simulink model "rti1401_program_controls_2018_test"  (R2017b)
settings: Solver=ode1  StartTime=0.0  StopTime=Inf  FixedStep=0.001  RelTol=1e-3  EnableMultiTasking=on
PreLoadFcn:
  | dataCar
  | load_vars
  | structAero
  | structEstimPar
  | structSensors
  | structSettings
PostLoadFcn:
  | , if any(exist('dsrtsu_mdlpostloadfcn', 'file') == [2, 3, 6]), try dsrtsu_mdlpostloadfcn('Execute', bdroot); catch fprintf('Error in PostLoadFcn (dsrtsu_mdlpostloadfcn) for model "%s":\n %s\n', bdroot, lasterr); end, end,
InitFcn:
  | dataCar
  | load_vars
  | structAero
  | structEstimPar
  | structSensors
  | structSettings
StartFcn:
  | dataCar
  | load_vars
  | structAero
  | structEstimPar
  | structSensors
  | structSettings
values from neighbouring files (symbols this model uses):
  Throttle_limits = [0.15, 0.90, 0.16, 0.92]    [load_vars.m]
undefined symbols (not defined in the file or in its folder): car, sensors
libraries: rtican x44, hdlsllib x32, simulink x8, rti1401lib_II_base x1
(part 11 of 11)

== matlab function rti1401_program_controls_2018_test/Processor/Control Systems/Traction Control ==
  data: sensors input; Torques output; settings input; estimPar input; torqueDistribution input; slipSet input; car parameter; TiTi2 output; error output; rpmSet output
function [Torques, TiTi2, error, rpmSet] = Traction(sensors, settings, estimPar, torqueDistribution, slipSet, car)

error =[0 0 0 0]';
persistent errorInt; if isempty(errorInt); errorInt=[0 0 0 0]'; end
persistent errorD; if isempty(errorD); errorD=[0 0 0 0]'; end
persistent errorPrev; if isempty(errorPrev); errorPrev=[0 0 0 0]'; end

%persistent wi_prev; if isempty(wi_prev); wi_prev=[0 0 0 0]'; end
%persistent SR_expected; if isempty(SR_expected); SR_expected=zeros(4, 8); end
%persistent wvi_prev; if isempty(wvi_prev); wvi_prev=[0 0 0 0]'; end

persistent TiPrev; if isempty(TiPrev); TiPrev=[0 0 0 0]'; end

persistent errorInt2; if isempty(errorInt2); errorInt2=[0 0 0 0]'; end
persistent Ti; if isempty(Ti); Ti=[0 0 0 0]'; end
persistent Ti2; if isempty(Ti2); Ti2=[0 0 0 0]'; end

rpmSet = [20000;20000;20000;20000];

if settings.TC == 1

    slipRatioTarget = slipSet;
    dist = estimPar.Fzi/sum(estimPar.Fzi);
    
    Kp = 100*dist*10;
    Ki = 40*dist*1000;
    Kd = 0*dist/100;
    Kv = 70/100;
    Mu = car.mu;
    
    Kp2 = 20*dist/1000;
    Ki2 = 40*dist/1000;
    
    %normal non linear torque control
    error = slipRatioTarget - estimPar.slip;
    
    errorInt = errorInt + error*car.dt;
    errorInt = min(max(errorInt,-0.001*[1;1;1;1]),0.003*[1;1;1;1]);
    errorD = min(max(errorD*0.1 + 0.9*(error - errorPrev)/car.dt,-25),25);
    lambdaD = Kp.*error + Ki.*errorInt + Kd.*errorD;
    Ti = lambdaD*car.tireInertia*max(estimPar.v,0)^Kv/car.tireRadius + sign(torqueDistribution).*estimPar.Fzi*(Mu)*car.tireRadius;
    Ti = Ti / car.gearRatio;
    
    %optimum seeking
    dFds = dFdsCalculator(estimPar.Fxi,estimPar.slip);
    error2 = dFds - 0;
    errorInt2 = errorInt2 + error2*car.dt;
    errorInt2 = min(max(errorInt2,-500*[1;1;1;1]),500*[1;1;1;1]);
    lambdaD2 = Kp2.*error2 + Ki2.*errorInt2;
    Ti2 = lambdaD2*car.tireInertia*max(estimPar.v,0)^Kv/car.tireRadius + sign(torqueDistribution).*estimPar.Fzi*(car.TC_mu)*car.tireRadius;
    Ti2 = Ti2 / car.gearRatio;
    
    for i=1:4
        if abs(error(i)) < 0.05
            Ti(i) = Ti2(i);
        end
    end
    
    if estimPar.v < 1/3.6
        %Ti = [80 80 180 180]';
        errorInt = [0 0 0 0]';
    end

    if sensors.throttle < 0.1
        errorInt = [0 0 0 0]';
    end
    
    lowerBoundary = TiPrev - 100/car.gearRatio;
    upperBoundary = TiPrev + 100/car.gearRatio;

    Ti = min(max(Ti,lowerBoundary),upperBoundary);
    
    TiPrev = Ti;
    errorPrev = error;
    
    Torques = Ti;
    for i=1:4
        if torqueDistribution(i) > 0
            Torques(i) = max(min(Torques(i),torqueDistribution(i)),0); 
        else
            Torques(i) = min(max(Torques(i),torqueDistribution(i)),0);
        end
    end
    
    
else
    Torques = torqueDistribution;
end

checkTorquemax = find((Torques > car.motor.Tmax)==1); %Limit torques to max torque
Torques(checkTorquemax)=car.motor.Tmax(checkTorquemax);



%wi_prev = sensors.wheelspeed;
%wvi_prev = sensors.wheelspeedi;

TiTi2 = [Ti;Ti2];

end

function [dFds] = dFdsCalculator(Fx,slipRatio)
N = 6;

persistent slipVector, if isempty(slipVector); slipVector = zeros(N,4); end
persistent FxVector, if isempty(FxVector); FxVector = zeros(N,4); end


FxVector(1,:) = Fx;
slipVector(1,:) = slipRatio;

dFds = [0;0;0;0];

for i=1:4
    p1 = polyfit(slipVector(:,i),FxVector(:,i),1);
    p2 = polyfit(FxVector(:,i),slipVector(:,i),1);
    
    rico1 = p1(1);
    rico2 = 1/p2(1);
    
    rico = sign(min(abs(rico1),abs(rico2)))*min(abs(rico1),abs(rico2));

    dFds(i) = max(min(rico,20000),-20000);
end

% shift list one
dummy = FxVector(1:N-1,:);
FxVector = [[0,0,0,0];dummy];
dummy = slipVector(1:N-1,:);
slipVector = [[0,0,0,0];dummy];

end

== matlab function rti1401_program_controls_2018_test/Processor/Control Systems/Yaw Rate Control ==
  data: sensors input; Mz output; settings input; estimPar input; car parameter; error output; actions output; rref output
function [Mz,error,actions,rref]= yawRateControl(sensors, settings, estimPar, car)
%Function that controls the moment around the z-axis
%INPUTS:
%OUTPUT: Moment of the car around Z-axis [Nm]

Mz = 0;
Mz_temp = 0;
rref = estimPar.rref;
error = 0;

wheelAngle = (sensors.wheelAngles(1)+sensors.wheelAngles(2))/2;

persistent Mz_memory; if isempty(Mz_memory); Mz_memory = 0; end
persistent errorInt; if isempty(errorInt); errorInt = 0; end
persistent errorDev; if isempty(errorDev); errorDev = 0; end
persistent prevError; if isempty(prevError); prevError = 0; end
persistent prevWheelAngle; if isempty(prevWheelAngle); prevWheelAngle = 0; end
persistent prevRref; if isempty(prevRref); prevRref = 0; end


error = estimPar.rref - sensors.yawRate;
errorInt = errorInt + error*car.dt;
errorInt = min(max(errorInt,-car.YRC.intLimit),car.YRC.intLimit);
errorDev = (error - prevError)/car.dt;
wheelAngleDev = (wheelAngle - prevWheelAngle)/car.dt;
rrefDev = (estimPar.rref - prevRref)/car.dt;

velocityGain = min(max(1 - (estimPar.v - car.YRC.changeVelocity)*car.YRC.slope,0),1);

Mz_temp = (car.YRC.Kp*error + car.YRC.Ki*errorInt + car.YRC.Kd*errorDev...
    +car.YRC.Ks*wheelAngleDev + car.YRC.Kr*rrefDev)*velocityGain;
Mz_temp = max(min(Mz_temp,car.YRC.maxValue),-car.YRC.maxValue);
Mz_memory=Mz_memory+Mz_temp;

P_Action = car.YRC.Kp*error;
I_Action = car.YRC.Ki*errorInt;
D_Action = car.YRC.Kd*errorDev;
steeringWheel_Action = car.YRC.Ks*wheelAngle;
yawRate_Action = car.YRC.Kr*estimPar.rref;

actions = [P_Action;I_Action;D_Action;steeringWheel_Action;yawRate_Action];
prevError = error;
prevWheelAngle = wheelAngle;
prevRref = estimPar.rref;



% if settings.YRC == 2
%     error = estimPar.rref - sensors.yawRate;
%     integral = integral + error*car.dt;
%     derivative = (error - prevError)/car.dt;
%
%     Mz_temp = car.YRC.Kp*error + car.YRC.Ki*integral + car.YRC.Kd*derivative...
%         +car.YRC.Ks*wheelAngle + car.YRC.Kr*estimPar.rref;
%     Mz_temp = max(min(Mz_temp,car.YRC.maxValue),-car.YRC.maxValue);
%
%     prevError = error;
% end



if settings.YRC ==1 %YRC enabled
    Mz = Mz_memory;
else %YRC disabled
    Mz = 0;
end

if car.YRC.minV > estimPar.v
    Mz = 0; %if speed is too low, don't activate yaw rate control
    errorInt = 0;
    prevError = 0;
end

rref=estimPar.rref;

== matlab function rti1401_program_controls_2018_test/Processor/Controller Settings1 ==
  data: settings output Bus: settingBus; sensors input; torqueMode input; Fsens input; TC input; Power input; Regen input; unlimitedFx input; effEstimation input; YRC input
function settings  = settingController(sensors,torqueMode,Fsens,TC,Power,Regen,unlimitedFx,effEstimation,YRC)

%TODO in test: bypass met P_elec controle, altijd tenzij P_elec sensor niet werkt

%==============%
%   Options    %
% 1 settings.torqueMode : 0,1,2
% 2 settings.Fsens : 0-100 in steps of 5
% 3 settings.TC : 0 or 1 (on/off)
% 4 settings.Power : 0-100 in steps of 10
% 5 settings.Regen : 0-30 in steps of 5
% 6 settings.unlimitedFx : 0 of 1
% 7 settings.effEstimation : 0,1,2
% 8 settings.YRC : 0 or 1 (on/off)
%==============%

error_detection = 1;
if any(sensors.errors == error_detection)
    if any(sensors.TCRE == error_detection)
        TC = 0;
    end
    torqueMode = uint8(0);
end

settings.Fxsens = 1;
settings.torqueMode = double(torqueMode);
settings.Fsens = double(Fsens);
settings.TC = TC;
settings.Power = double(Power)/16;
settings.Regen = double(Regen);
settings.unlimitedFx = unlimitedFx;
settings.effEstimation = effEstimation;
settings.YRC = YRC;

== matlab function rti1401_program_controls_2018_test/Processor/Decisive Logic Block/MATLAB Function ==
  data: torqueController input; torques output; rpmController input; torqueBypass input; rpmBypass input; rpmRef output; settings input
function [torques,rpmRef]= DLB(torqueController,rpmController,torqueBypass,rpmBypass,settings)

torques = [0;0;0;0];
rpmRef = [0;0;0;0];

if settings.torqueMode == 0
    
    torques = settings.Power*torqueBypass;
    rpmRef = rpmBypass;
    
else
    
    torques = settings.Power*torqueController;
    rpmRef = rpmController;
    
end

== matlab function rti1401_program_controls_2018_test/Processor/Vehicle Estimated Parameters/Extended Kalman Filter ==
  data: F_KF input; States output; H_KF input; y_meas input; y_pred input; R_beta_lin input; Q_Cy input; sensors input; P_est input; P_est output
function [States, P_est]  = EKF(F_KF,H_KF,y_meas, y_pred, R_beta_lin, Q_Cy, sensors, P_est)
 
 %% Initialization of global variables %%
 
global vy_g psi_dot_g vx_g Cf_g Cr_g P_est_glob

delta = (sensors.wheelAngles(1)+sensors.wheelAngles(2))/2;
 %% Calculation partitioned F-matrix %%
F = F_KF;
 
 %% Calculation partitioned H-matrix %%
H = H_KF;

% ============================== Parameters ===============================
% number of observable states
n_xo = 3;
% number of unobservable states
n_xu = 2;
% total number of states
n_x = n_xo + n_xu;
% number of system inputs
n_u = 2;
% number of measurements
n_y = 7;
% covariance of modeled process noise

Q_Cyf = Q_Cy;
Q_Cyr = Q_Cy;
Q_vy = 1*10^(-6);
Q_psi_dot = 1*10^(-6);
Q_vx = 1*10^(-4);

Q_oo = [Q_vy, 0, 0;
    0, Q_psi_dot, 0;
    0, 0, Q_vx];

Q_uu = [Q_Cyf, 0;
     0, Q_Cyr];
 
Q_model = [Q_vy, 0, 0, 0, 0;
    0, Q_psi_dot, 0, 0, 0;
    0, 0, Q_vx, 0, 0;
    0, 0, 0, Q_Cyf, 0;
    0, 0, 0, 0, Q_Cyr];

% covariance of measurement noise

R_psi_dot = 2.4*10^(-7);
R_ay = 2.5*10^(-3);
R_vxfl = 1*10^(-5);
R_vxfr = 1*10^(-5);
R_vxrl = 1*10^(-5);
R_vxrr = 1*10^(-5);
R_beta = R_beta_lin;
R_model = [R_psi_dot, 0, 0, 0, 0, 0, 0;
    0, R_ay, 0, 0, 0, 0, 0;
    0, 0, R_vxfl, 0, 0, 0, 0;
    0, 0, 0, R_vxfr, 0, 0, 0;
    0, 0, 0, 0, R_vxrl, 0, 0;
    0, 0, 0, 0, 0, R_vxrr, 0;
    0, 0, 0, 0, 0, 0, R_beta];
% covariance of simulated process noise
Q_sim = [Q_vy, 0, 0, 0, 0;
    0, Q_psi_dot, 0, 0, 0;
    0, 0, Q_vx, 0, 0;
    0, 0, 0, Q_Cyf, 0;
    0, 0, 0, 0, Q_Cyr];
% covariance of simulated measurement noise
R_sim = [R_psi_dot, 0, 0, 0, 0, 0, 0;
    0, R_ay, 0, 0, 0, 0, 0;
    0, 0, R_vxfl, 0, 0, 0, 0;
    0, 0, 0, R_vxfr, 0, 0, 0;
    0, 0, 0, 0, R_vxrl, 0, 0;
    0, 0, 0, 0, 0, R_vxrr, 0;
    0, 0, 0, 0, 0, 0, R_beta];
% initial state
x0 = [0; 0; 0; car.Cf_lin; car.Cr_lin];
% initial state estimate
% x_est0 = [0; 0; 0; car.Cf_lin; car.Cr_lin];
% feedback values
% kx = 0.1;
% ky = 0.1;
% kt = 0.1;

% ==================== Simulation Preparation ===========================

if isempty(P_est_glob) == 1
    states = x_0;
    P_est= eye(n_x)*10^(-4);
    
else
    states = [vy_g, psi_dot_g, vx_g, Cf_g, Cr_g];
    
end
       
inputs_EKF = [delta; sensors.ax];

P_est_pre_tot = zeros(n_x, n_x);

P_est_post_tot = zeros(n_x, n_x);


% feedback matrix
% K = [kx,  0,  0;
%       0, ky, kt];


% ==================== Kalman prediction step ===========================

states = f_est(states, inputs_EKF, car.dt);

P_est_pre = F*P_est*F^(-1)+Q_model;

%P_est_pre_oo = A*P_est_post(:,:,i-1)*A' + Q_mod;
%      P_est(:,:,i) = A*P_est(:,:,i-1)*A';

% ==================== Kalman correction step ===========================

nu = y_meas - y_pred;
%      nu(:,i) = y(:,i) - h(x_est(:,i));
S = H*P_est_pre*H' + R_model;
%      S(:,:,i) = C*P_est(:,:,i)*C';
K = P_est_pre*H'/S;

states = states + K*nu;
P_est_post = (eye(n_x)-K*H)*P_est_pre;

States.vy_g = states(1);
States.psi_dot_g = states(2);
States.vx_g = states(3);
States.Cf_g = states(4);
States.Cr_g = states(5);

P_est = P_est_post;
P_est_glob = P_est;

% %     Control law
% u(:,i) = u_ref(:,i);
% %     err_loc(:,i) = local_error(x_ref(:,i), x_est(:,i));
% %     u(:,i) = u_ref(:,i) + K*err_loc(:,i);

end

== matlab function rti1401_program_controls_2018_test/Processor/Vehicle Estimated Parameters/Covariantie ==
  data: sensors input; R_beta_lin output; yawrate_lin input; Q_Cy output; car parameter
function [R_beta_lin, Q_Cy] = Covariantie(sensors,yawrate_lin, car)
if (abs(sensors.yawRate)-abs(yawrate_lin)) > car.e_max && abs(sensors.yawRate)>0 && abs(yawrate_lin)>0
    
    global counter
    
    if isempty(counter)
        counter = 0
    end
    
    counter = counter + 1;
    array_dev_yawrate = zeros(1,1.5*(1/car.dt));
    delta = (sensors.wheelAngles(1)+sensors.wheelAngles(2))/2;
    % Q_Cyi wordt hoog gezet, net als R_beta_lin, en hoe groter het verschil, hoe groter de 
    % onnauwkeurigheid zal worden (dev_ya wrate = e uit de paper)
    dev_yawrate = abs(sensors.yawRate)-abs(yawrate_lin);
    
    if counter < 1.5*(1/car.dt)
        array_dev_yawrate(counter) = dev_yawrate;
        
    else
        for k = 2:length(array_dev_yawrate)
            array_dev_yawrate(k-1)=array_dev_yawrate(k);
        end
        array_dev_yawrate(length(array_dev_yawrate)) = dev_yawrate;
    end
    
    dev_yawrate_max = max(array_dev_yawrate);
    % We gaan best een referentiewaarde nemen voor Q_Cyi voor het geval het
    % verschil < car.e_max
    Q_Cy0 = car.Q_Cyref*log(9*(delta/car.delta_max)+1);%functie nog aanpasbaar
    R_beta_lin0 = car.R_beta_linref*log(8*(delta/car.delta_max)+2);
    
    
    
    Q_Cy = Q_Cy0 + 500*dev_yawrate_max^2;
    R_beta_lin = R_beta_lin0 + (5*array_dev_yawrate)^4;
    
else
    delta = (sensors.wheelAngles(1)+sensors.wheelAngles(2))/2;
    Q_Cy0 = car.Q_Cyref*log(9*(delta/car.delta_max)+1);%functie nog aanpasbaar
    R_beta_lin0 = car.R_beta_linref*log(8*(delta/car.delta_max)+2);
    Q_Cy = Q_Cy0;
    R_beta_lin = R_beta_lin0;
end

end

== matlab function rti1401_program_controls_2018_test/Processor/Vehicle Estimated Parameters/Estimation Parameters ==
  data: States input; estimPar output; car parameter; sensors parameter; Fzi input; Fyi input; Fxi input; alpha input; eff input; rref input
function estimPar  = estimation_par(States, car, sensors, Fzi, Fyi, Fxi, alpha, eff, rref)
%% Forming "States_final" %%

estimPar.vy_g = States.vy_g;
estimPar.psi_dot_g = States.psi_dot_g;
estimPar.vx_g = States.vx_g;
estimPar.Cf_g = States.Cf_g;
estimPar.Cr_g = States.Cr_g;
estimPar.Fzi=Fzi;
estimPar.Fxi=Fxi;
estimPar.Fyi=Fyi;
estimPar.alpha_f = alpha.f;
estimPar.alpha_r = alpha.r;
estimPar.eff = eff;
estimPar.rref = rref;
end

== matlab function rti1401_program_controls_2018_test/Processor/Vehicle Estimated Parameters/Fx_estimation ==
  data: States input; Fxi output; car parameter; sensors parameter
function Fxi  = Fx_estimation(States,car, sensors)

%OPM: gearratio zit al verwerkt in sensors.torque (= wheelTorque)

persistent wheelspeedPrev; if isempty(wheelspeedPrev); wheelspeedPrev = [0 ;0 ;0 ;0]; end
persistent inertia; if isempty(inertia); inertia = car.tireInertia; end
if isempty(States.vx_g); States.vx_g =0;end
wheelspeed = sensors.wheelspeed;
alpha = (wheelspeed - wheelspeedPrev)/car.dt;

%wheelTorque = car.gearRatio*sensors.torque -(car.motor.Inertia*car.gearRatio^2 - car.tireInertia)*alpha;
%to be used if only motor torque is known (real scenario)

%Fxi_est = (wheelTorque - alpha*inertia)/car.tireRadius;
Fxi_est = (sensors.torque - alpha*inertia)/car.tireRadius;
%Fxi_est = (sensors.torque)/car.tireRadius;

Fx_tot = sensors.ax*car.mass + 0.5*car.rhoAir*States.vx_g^2*car.Cd*car.AFront;
Fxi = Fxi_est;




wheelspeedPrev=wheelspeed;
inertiaOut = inertia;
end

== matlab function rti1401_program_controls_2018_test/Processor/Vehicle Estimated Parameters/Fy_distribution ==
  data: States input; Fyi output; car parameter; sensors parameter; Fzi input; alpha output
function [Fyi,alpha] = Fy_distribution(States,car, sensors, Fzi)

%% Calculation sideslip angles of the wheels %%
delta = (sensors.wheelAngles(1)+sensors.wheelAngles(2))/2;
alpha.f = -((States.vy_g + car.lf*States.psi_dot_g)/(States.vx_g)) + delta;
alpha.r = -((States.vy_g - car.lr*States.psi_dot_g)/(States.vx_g));

%% Calculation OF Lateral forces (Bycicle model) %%
F_yf = 2*States.Cf_g*alpha.f;
F_yr = 2*States.Cr_g*alpha.r;

%% Distribution of lateral force on left and right tire by using the normal force distribution %%


%Use of a scale factor 

FzRatioFront = [Fzi(1); Fzi(2)]./sum(Fzi(1:2));
FzRatioRear = [Fzi(3); Fzi(4)]./sum(Fzi(3:4));


scaleFactorFy = 0.7;
FyFrontDiff = (FzRatioFront(1) - FzRatioFront(2))*scaleFactorFy/2;
Fy_FL = F_yf/2 + FyFrontDiff* F_yf;
Fy_FR = F_yf/2 - FyFrontDiff* F_yf;
FyRearDiff = (FzRatioRear(1) - FzRatioRear(2))*scaleFactorFy/2;
Fy_RL = F_yr/2 + FyRearDiff* F_yr;
Fy_RR = F_yr/2 - FyRearDiff* F_yr;
    
Fyi=[Fy_FL;Fy_FR;Fy_RL;Fy_RR];

== matlab function rti1401_program_controls_2018_test/Processor/Vehicle Estimated Parameters/Fz_estimation ==
  data: States input; Fzi output; car parameter; sensors parameter; aero output
function [Fzi, aero] = Fz_estimation(States,car, sensors)

%% Calculation of Normal Forces F_zi %%

if isempty(States.vx_g); States.vx_g =0;end
%Dynamical loads 
%Without taking suspension into account

aero.FD = 0.5*car.Cd*car.AFront*car.rhoAir*States.vx_g^2; %drag force, pointing rearward [N]
aero.FL = 0.5*car.Cl*car.AFront*car.rhoAir*States.vx_g^2; %lift force, pointing upward [N]
aero.lever_FD = [-0.1;0.1]; %distance from the COG to the point of application of the drag [m]
aero.lever_FL = [-0.1;0.1]; %distance from the COG to the point of application of the lift [m]

FFA = car.g*car.mass*car.lr/car.wb - (car.h/car.wb)*(car.mass*sensors.ax) - ...
    aero.FD*((car.h+aero.lever_FD(2))/car.wb) - ...
    aero.FL*((car.lr-aero.lever_FL(1))/car.wb); %dyn load Front Axle
FRA = car.g*car.mass*car.lf/car.wb + (car.h/car.wb)*(car.mass*sensors.ax) + ...
    aero.FD*((car.h+aero.lever_FD(2))/car.wb) - ...
    aero.FL*((car.lf+aero.lever_FL(1))/car.wb); %dyn load Rear Axle


FFL = FFA/2 - (car.h/(2*car.tw))*(car.mass*sensors.ay);
FFR = FFA/2 + (car.h/(2*car.tw))*(car.mass*sensors.ay);
FRL = FRA/2 - (car.h/(2*car.tw))*(car.mass*sensors.ay);
FRR = FRA/2 + (car.h/(2*car.tw))*(car.mass*sensors.ay);


Fzi = [FFL;FFR;FRL;FRR];

== matlab function rti1401_program_controls_2018_test/Processor/Vehicle Estimated Parameters/MATLAB Function ==
  data: eff output; settings input; car parameter; sensors input
function eff = Efficiency(settings,car, sensors)
%P_elec * eff = P_mech

persistent effTemp; if isempty(effTemp); effTemp = 0.7; end
persistent errorInt; if isempty(errorInt); errorInt = 0; end

Pmax = car.Pmax - car.PC.safetyMargin; %[W]

P_mech = sum(sensors.torque.*sensors.wheelspeed); %*car.gearRatio
P_elec = sensors.P_elec;
ratio = 0.2;

if settings.effEstimation == 1
    
    if P_elec > 1
        effCalc = P_mech/P_elec;
        effTemp = effTemp*ratio + (1-ratio)*min(max(effCalc,car.PC.minEff),car.PC.maxEff);
        
    elseif P_elec < 1
        effCalc = P_elec/min(P_mech,-1);
        effTemp = effTemp*ratio + (1-ratio)*min(max(effCalc,car.PC.minEff),car.PC.maxEff);
        
        
        %mogelijkheid tot uitbreiding: Pmax variable ifv van batterij voor tijdens
        %indurance
    end
    
end

if settings.effEstimation == 2
    
    if P_elec > Pmax*0.3 && sensors.throttle > 0 % only positive power limit
        
        error = (Pmax - P_elec)/Pmax;
        if error < 0 % P_elec > Pmax
            error = error*2;
        end
        
        errorInt = errorInt + error*car.dt;
        errorInt = max(min(errorInt,0.2),-0.2);
        
        dEff = car.PC.Kp*error + car.PC.Ki*errorInt; %more fitting variable name would be powerReductionFactor as this is not anymore an efficiency as Pelec * eff = Pmech
        %make car.PC.Kp velocity dependend?
        
        effTemp = max(min(effTemp + dEff,car.PC.maxEff),car.PC.minEff);
        
    else
        if P_elec > 5000
            eta = P_mech/P_elec;
            effTemp = effTemp*ratio+(1-ratio)*min(max(eta,car.PC.minEff),car.PC.maxEff);
        elseif P_elec < -5000
            eta = P_elec/min(P_mech,-1);
            effTemp = effTemp*ratio+(1-ratio)*min(max(eta,car.PC.minEff),car.PC.maxEff);
        end
        
    end
    
else
    effTemp = effTemp;
    
end


eff = effTemp;
effnotcontrolled = P_mech/P_elec;

== matlab function rti1401_program_controls_2018_test/Processor/Tire model//friction coefficient estimation/MATLAB Function ==
  data: mu input; estimParExtended output; estimPar input
function estimParExtended  = estimParExtension(mu, estimPar)

estimParExtended.vy_g = estimPar.vy_g;
estimParExtended.psi_dot_g = estimPar.psi_dot_g;
estimParExtended.vx_g = estimPar.vx_g;
estimParExtended.Cf_g = estimPar.Cf_g;
estimParExtended.Cr_g = estimPar.Cr_g;
estimParExtended.Fzi=estimPar.Fzi;
estimParExtended.Fxi=estimPar.Fxi;
estimParExtended.Fyi=estimPar.Fyi;
estimParExtended.alpha_f = estimPar.alpha.f;
estimParExtended.alpha_r = estimPar.alpha.r;
estimParExtended.eff = estimPar.eff;
estimParExtended.mu = mu;
estimParExtended.rref = estimPar.rref;

== matlab function rti1401_program_controls_2018_test/Processor/Vehicle Estimated Parameters/Slip Ratio ==
  data: States input; slip_ratio output; car parameter; sensors parameter
function slip_ratio = slip_ratio(States, car, sensors)

if isempty(States.vx_g); States.vx_g =0;end
yawRate = [0;0;States.psi_dot_g];
dist = [car.lf   -car.lf   car.lr   -car.lr;
        car.tl/2 -car.tl/2 car.tr/2 -car.tr/2;
        0        0         0        0];
omegaR = sensors.wheelspeed*car.tireRadius;

%Thesis BreyneMeulemans eq 3.20-3.22
v_xcomp = zeros(4,1);
d = sensors.wheelAngles;
for i=1:4
    R = [cos(d(i)) sin(d(i)) 0;
        -sin(d(i)) cos(d(i)) 0;
        0          0         1];
    v_rel = cross(yawRate,dist(:,i));
    v_abs = v_rel + [States.vx_g;0;0];
    v_ab2 = R*v_abs;
    v_xcomp(i) = v_ab2(1);
end

if sensors.ax > 0
    slip_ratio = (omegaR - v_xcomp)./omegaR;
elseif sensors.ax < 0
    slip_ratio = (omegaR - v_xcomp)./v_xcomp;
else
    slip_ratio = [0;0;0;0];
end
end

== matlab function rti1401_program_controls_2018_test/Processor/Vehicle Estimated Parameters/Yawrate Reference ==
  data: rref output; States input; car parameter; sensors parameter
function rref = yawRateRef(States, car, sensors)
if isempty(States.vx_g); States.vx_g =0;end
%Ackermann
wheelAngle = (sensors.wheelAngles(1)+sensors.wheelAngles(2))/2;
rref = wheelAngle*States.vx_g/car.wb;

== matlab function rti1401_program_controls_2018_test/Processor/Vehicle Estimated Parameters/States_matrix_generation ==
  data: estimPar input; States_matrix_front output; N_est input; Fy_est input; Fx_est input; States_matrix_rear output; slip_ratio input
function [States_matrix_front, States_matrix_rear] = States_matrix_gen(estimPar, N_est, Fy_est, Fx_est, slip_ratio)

global counter_mat 

if isempty(counter_mat)
    counter_mat = 0
end

counter_mat = counter_mat+1;
States_matrix_front = zeros(3,1);
States_matrix_rear = zeros(3,1);
slip_ratio_front = (slip_ratio(1)+slip_ratio(2))/2;
slip_ratio_rear = (slip_ratio(3)+slip_ratio(4))/2;

while counter_mat < 1000
    States_matrix_front(:,counter_mat) = [estimPar.alpha_f, N_est.f, Fy_est.f, slip_ratio_front, Fx_est.f];
    States_matrix_rear(:,counter_mat) = [estimPar.alpha_r, N_est.r, Fy_est.r, slip_ratio_rear, Fx_est.r];
    
end
end

== matlab function rti1401_program_controls_2018_test/Processor/Vehicle Estimated Parameters/Normal forces calculation ==
  data: States input; N_est output; Fy_est output; car parameter; sensors parameter; Fxi input; Fx_est output
function [N_est, Fy_est, Fx_est] = N_F_calc(States, car, sensors, Fxi)

N_est.f = (car.mass)*9.81*((car.lr)/(car.lr+car.lf))- (sensors.ax)*(car.mass)*(car.h);
N_est.r = (car.mass)*9.81*((car.lr)/(car.lr+car.lf))+ (sensors.ax)*(car.mass)*(car.h);

Fy_est.f = 2*(States.Cf_g)*(alpha.f);
Fy_est.r = 2*(States.Cf_r)*(alpha.r);

Fx_est.f = Fxi(1)+Fxi(2);
Fx_est.r = Fxi(3)+Fxi(4);

== matlab function rti1401_program_controls_2018_test/Processor/Vehicle Estimated Parameters/MATLAB Function1 ==
  data: States input; alpha_wheels output; sensors parameter; car parameter
function alpha_wheels  = v_alpha_decomp(States, sensors, car)

%% Calculation vx on each independant wheel %%

vx_wheels.fl = (States.vx_g - States.psi_dot_g*(car.tf/2))*cos(sensors.wheelAngles(1)) + ...
        States.psi_dot_g*(car.lf)*sin(sensors.wheelAngles(1));
    
vx_wheels.fr = (States.vx_g + States.psi_dot_g*(car.tf/2))*cos(sensors.wheelAngles(2)) + ...
        States.psi_dot_g*(car.lf)*sin(sensors.wheelAngles(2));
    
vx_wheels.rl = (States.vx_g - States.psi_dot_g*(car.tr/2));
    
vx_wheels.rr = (States.vx_g + States.psi_dot_g*(car.tr/2));

%% Calculation vy on each independant wheel %%

vy_wheels.fl = (States.vy_g + States.psi_dot_g*(car.lf))*cos(sensors.wheelAngles(1)) + ...
        States.psi_dot_g*(car.tf/2)*sin(sensors.wheelAngles(1));
    
vy_wheels.fr = (States.vy_g - States.psi_dot_g*(car.tf/2))*sin(sensors.wheelAngles(2)) + ...
        States.psi_dot_g*(car.lf)*cos(sensors.wheelAngles(2));
    
vy_wheels.rl = (States.vy_g - States.psi_dot_g*(car.lr));
    
vy_wheels.rr = (States.vy_g - States.psi_dot_g*(car.lr));

%% Calculation alpha's on each independant wheel %%

alpha_wheels.fl = atan2(vy_wheels.fl,vx_wheels.fl);
alpha_wheels.fr = atan2(vy_wheels.fr,vx_wheels.fr);
alpha_wheels.rl = atan2(vy_wheels.rl,vx_wheels.rl);
alpha_wheels.rr = atan2(vy_wheels.rr,vx_wheels.rr);

== matlab function rti1401_program_controls_2018_test/Processor/Tire model//friction coefficient estimation/Tire model estimation ==
  data: States_matrix_front input; Settings_extended output; States_matrix_rear input; Settings input; Magic_tire_param output
function [Settings_extended, Magic_tire_param] ...
    = Est_tire_model(States_matrix_front, States_matrix_rear, Settings)


if length(States_matrix_front) == 1000   % Indien we sampelen op 100Hz krijgen we dit in 10s
                                         % wat ongeveer de duur is van het
                                         % skidpad event
    p0 = tire_model_est_test(States_matrix_front, States_matrix_rear);
    Settings.act_TV = 1;
end

% The following if-statement is ONLY used when the tire model is
% determined. In the normal case, the driver decides wheter or not he
% activates the TV-mode. When the tire model will be determined (probably
% during skidpad event), following if-statement simply overrules the
% decision of the driver. This means, in the first run of the skidpad
% event, the driver won't be able to use the TV-mode.

if length(States_matrix_front) > 1000
    Settings.torqueMode = 1;
else
    Settings.torqueMode = 0;
end

Settings_extended = Settings;
Magic_tire_param.front_x = p0.front_x;
Magic_tire_param.front_y = p0.front_y;
Magic_tire_param.rear_x = p0.rear_x;
Magic_tire_param.rear_y = p0.rear_y;

== matlab function rti1401_program_controls_2018_test/Processor/Tire model//friction coefficient estimation/friction frank test   ==
  data: mu output; estimPar input; Magic_tire_param input; Fzi input; slip_ratio input; alpha_wheels input; States_matrix_front input
function mu  = frictionfrank(estimPar,Magic_tire_param,Fzi,slip_ratio, alpha_wheels, States_matrix_front)
%This function calculates an estimate for the maximum friction coefficient
%by comparing the estimated forces with the forces calculated using the
%Dugoff tire model for a certain side slip angle and slip ratio. The forces
%are calculated for a range of mu values, and the mu for which the forces
%deviate the least (rms) is chosen as the instantaneous mu value.
if length(States_matrix_front) >= 1000
    mu = [0.05;0.05;0.05;0.05];
    rms1 = [0;0;0;0];
    rms2 = [0;0;0;0];

    alpha_mu = [alpha_wheels.fl, alpha_wheels.fr, alpha_wheels.rl, alpha_wheels.rr];

    p0x = [Magic_tire_param.front_x; Magic_tire_param.front_x; ...
    Magic_tire_param.rear_x;Magic_tire_param.rear_x];
    p0y = [Magic_tire_param.front_y; Magic_tire_param.front_y; ...
        Magic_tire_param.rear_y;Magic_tire_param.rear_y];

    for i=1:1:4
        F_xd = Fzi(i)*p0x(i,3)*sin(p0x(i,2)*atan(p0x(i,1)*(1-p0x(i,4))*slip_ratio(i) + ...
            atan(p0x(i,1)*slip_ratio(i))));
        F_yd = Fzi(i)*p0y(i,3)*sin(p0y(i,2)*atan(p0y(i,1)*(1-p0y(i,4))*alpha_mu(i) + ...
            atan(p0y(i,1)*alpha_mu(i))));
   
        rms1(i) = sqrt((estimPar.Fxi(i)-F_xd)^2+(estimPar.Fyi(i)-F_yd)^2);
    end
    for i=1:1:4
        for mu1=0.1:0.05:1
            F_xd1 = Fzi(i)*p0x(i,3)*sin(p0x(i,2)*atan(p0x(i,1)*(1-p0x(i,4))*slip_ratio(i) + ...
                atan(p0x(i,1)*slip_ratio(i))));
            F_yd1 = Fzi(i)*p0y(i,3)*sin(p0y(i,2)*atan(p0y(i,1)*(1-p0y(i,4))*alpha_mu(i) + ...
                atan(p0y(i,1)*alpha_mu(i))));
            rms2(i) = sqrt((estimPar.Fxi(i)-F_xd1)^2+(estimPar.Fyi(i)-F_yd1)^2);
            if rms2(i) < rms1(i)
                mu(i) = mu1;
                rms1(i) = rms2(i);
            end
        end
    
    end
end

end

== matlab function rti1401_program_controls_2018_test/Processor/Tire model//friction coefficient estimation/Magic tire param workspace ==
  data: Magic_tire_param input; Magic_Tire_Param_front_x output; Magic_Tire_Param_front_y output; Magic_Tire_Param_rear_x output; Magic_Tire_Param_rear_y output
function [Magic_Tire_Param_front_x, Magic_Tire_Param_front_y, Magic_Tire_Param_rear_x,...
    Magic_Tire_Param_rear_y] = MTF_workspace(Magic_tire_param)

Magic_Tire_Param_front_x = Magic_tire_param.front_x;
Magic_Tire_Param_front_y = Magic_tire_param.front_y;
Magic_Tire_Param_rear_x = Magic_tire_param.rear_x;
Magic_Tire_Param_rear_y = Magic_tire_param.rear_y;

end

== matlab function rti1401_program_controls_2018_test/Processor/Sensors ==
  data: ax input; sensors output Bus: sensorBus size=1; ay input; yawRate input; steeringAngle input; steerAngleFL input; steerAngleFR input; throttle input; brake input; wheelspeed_FL input; wheelspeed_FR input; wheelspeed_RL input; wheelspeed_RR input; torqueFL input; torqueFR input; torqueRL input; torqueRR input; P_elec input; car parameter
function sensors = sensors(ax,ay,yawRate,steeringAngle,steerAngleFL,steerAngleFR, throttle,brake,wheelspeed_FL,wheelspeed_FR,wheelspeed_RL,wheelspeed_RR,torqueFL,torqueFR,torqueRL,torqueRR,P_elec,car)

sensors.ax = double(ax);
if ax > 50 || ax < -50
    sensors.ax_error = 1;
else
    sensors.ax_error = 0;
end
sensors.ay = double(ay);
if ay > 50 || ay < -50
    sensors.ay_error = double(1);
else
    sensors.ay_error = double(0);
end

sensors.wheelspeed = double([wheelspeed_FL;wheelspeed_FR;wheelspeed_RL;wheelspeed_RR]);
if wheelspeed_FL > 20000 || wheelspeed_FL < -1000
    sensors.wheelspeed_error = 1;
elseif wheelspeed_FR > 20000 || wheelspeed_FR < -1000
    sensors.wheelspeed_error = 1;
elseif wheelspeed_RL > 20000 || wheelspeed_RL < -1000
    sensors.wheelspeed_error = 1;
elseif wheelspeed_RR > 20000 || wheelspeed_RR < -1000
    sensors.wheelspeed_error = 1;
else
    sensors.wheelspeed_error = 0;
end
sensors.wheelspeed = double(sensors.wheelspeed./60.*2.*pi); %rpm to rad/s

sensors.yawRate = double(yawRate);
if yawRate > 50 || yawRate < -50
    sensors.yawRate_error = 1;
else
    sensors.yawRate_error = double(0);
end

sensors.steerAngle = double(steeringAngle);
if steeringAngle > 300 || steeringAngle < -300
    sensors.steerAngle_error = 1;
else
    sensors.steerAngle_error = double(0);
end

sensors.wheelAngles = double([steerAngleFL;steerAngleFR;0;0]);
if steerAngleFL > 40 || steerAngleFL < -40
    sensors.wheelAngle_error = 1;
elseif steerAngleFR > 40 || steerAngleFR < -40
    sensors.wheelAngle_error = 1;
else
    sensors.wheelAngle_error = 0;
end

sensors.throttle = double(throttle);
if throttle > 100 || throttle < 0
    sensors.throttle_error = double(1);
else
    sensors.throttle_error = 0;
end

sensors.brake = double(brake);
if brake > 100 || brake < 0
    sensors.brake_error = double(1);
else
    sensors.brake_error = 0;
end

sensors.torque = double([torqueFL;torqueFR;torqueRL;torqueRR]);
if torqueFL > 25 || torqueFL < -25
    sensors.torque_error = 1;
elseif torqueFR > 25 || torqueFR < -25
    sensors.torque_error = 1;
elseif torqueRL > 25 || torqueRL < -25
    sensors.torque_error = 1;
elseif torqueRR > 25 || torqueRR < -25
    sensors.torque_error = 1;
else
    sensors.torque_error = 0;
end

sensors.P_elec = double(P_elec);
if P_elec > 160 || P_elec < 0
    sensors.P_elec_error = 1;
else
    sensors.P_elec_error = 0;
end

sensors.errors = [sensors.ax_error;sensors.ay_error;sensors.wheelspeed_error;...
    sensors.yawRate_error;sensors.wheelAngle_error;sensors.throttle_error;...
    sensors.brake_error;sensors.torque_error;sensors.P_elec_error];
sensors.TCRE = [sensors.ax_error;sensors.ay_error;sensors.wheelspeed_error;...
    sensors.throttle_error;sensors.brake_error;sensors.torque_error;...
    sensors.P_elec_error];
    %Traction Control Relevant Errors

AccVector = [sensors.ax;sensors.ay;0]+cross([0;0;sensors.yawRate],...
    [car.distECUx;car.distECUy;car.distECUz])+cross([0;0;sensors.yawRate],...
    cross([0;0;sensors.yawRate],[car.distECUx;car.distECUy;car.distECUz]));
sensors.ax = AccVector(1);
sensors.ay = AccVector(2);
    %Acceleration transformation
    %Thesis BreyneMeulemans eq 3.2

== matlab function rti1401_program_controls_2018_test/Processor/Ackermann Arno ==
  data: x input; thetaL output; thetaR output
function [thetaL, thetaR]= ackermann(x)
%x is de rack travel in mm
%+ als rack naar rechts beweegt van achter de wagen bekeken
%- als rack naar links beweegt van achter de wagen bekeken

thetaL=-2*(10^-9)*(x^6)+8*(10^-8)*(x^5)+9*(10^-7)*(x^4)+3*(10^-5)*(x^3)-0.0049*(x^2)+1.0437*x+0.0254;
%thetaL is hoeverdraaiing van linker wiel in °
%-hoek is draaien naar links van boven de wagen bekeken
%+hoek is draaien naar rechts van boven de wagen bekeken

thetaR=2*(10^-9)*(x^6)+8*(10^-8)*(x^5)-9*(10^-7)*(x^4)+3*(10^-5)*(x^3)+0.0049*(x^2)+1.0437*x-0.0254;
%thetaR is hoekverdraaiing van rechter wiel in °
%-hoek is draaien naar links van boven de wagen bekeken
%+hoek is draaien naar rechts van boven de wagen bekeken

end
